simulink model "quadrotor_control"  (R2017b)
settings: Solver=FixedStepAuto  StartTime=0.0  StopTime=5  FixedStep=0.1  MinStep=0.02  RelTol=1e-3  AbsTol=0.001  EnableMultiTasking=on
PreLoadFcn:
  | m=0;
libraries: simulink x9
settings Model: Creator=GPH_PC  LastModifiedBy=dell
settings SolverCC: InitialStep=0.03
settings DataIOCC: LimitDataPoints=on  SaveFormat=Array
settings OptimizationCC: LifeSpan=inf
settings DebuggingCC: SolverPrmCheckMsg=warning  SFUnexpectedBacktrackingDiag=warning  SFNoUnconditionalDefaultTransitionDiag=warning  SFExecutionAtInitializationDiag=none
settings HardwareCC: ProdBitPerPointer=32  ProdBitPerSizeT=32  ProdBitPerPtrDiffT=32  ProdLargestAtomicFloat=None  ProdIntDivRoundTo=Undefined  ProdEndianess=Unspecified  ProdWordSize=32  ProdHWDeviceType=32-bit Generic
settings ModelReferenceCC: PropagateSignalLabelsOutOfModel=off
settings CodeAppCC: StateflowObjectComments=on
settings GRTTargetCC: TargetLangStandard=C89/C90 (ANSI)  GeneratePreprocessorConditionals=Disable all
settings ConfigComp: CovMetricSettings=dw  CovHtmlReporting=on  CovSaveCumulativeToWorkspaceVar=on  CovSaveSingleToWorkspaceVar=on  CovExternalEMLEnable=off  CovSFcnEnable=off

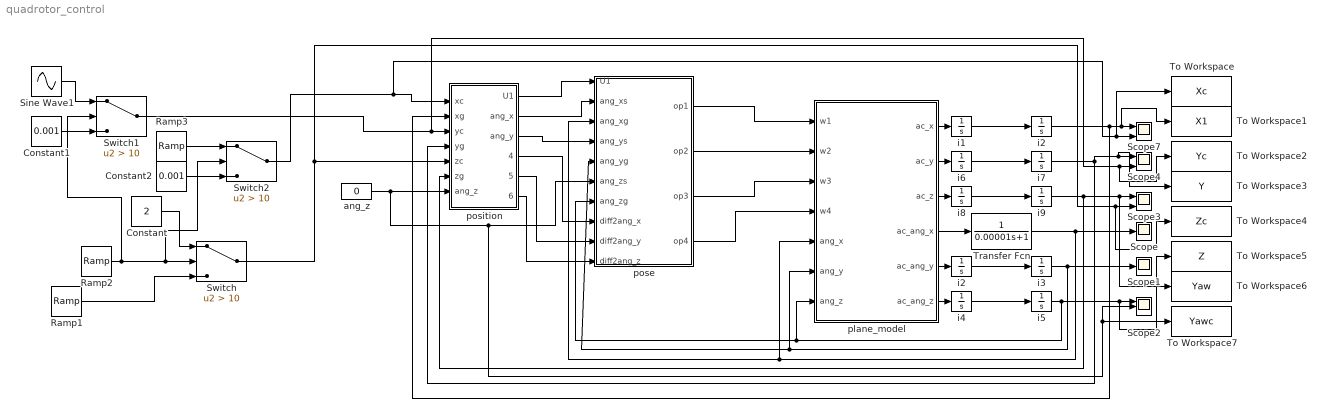
== system quadrotor_control ==
  " i2" : Integrator
  Constant : Constant  Value=2
  Constant1 : Constant  Value=0.001
  Constant2 : Constant  Value=0.001
  Ramp1 : simulink/Sources/Ramp  slope=0.2  start=0  X0=0
  Ramp2 : simulink/Sources/Ramp  slope=1  start=0  X0=0
  Ramp3 : simulink/Sources/Ramp  slope=1  start=0  X0=0
  Scope : Scope
  Scope1 : Scope
  Scope{2..4,7} (4 alike) : Scope  NumInputPorts=3
  Sine Wave1 : Sin  Amplitude=3  SampleTime=0
  Switch : Switch  Criteria=u2 > Threshold  Threshold=10
  Switch1 : Switch  Criteria=u2 > Threshold  Threshold=10
  Switch2 : Switch  Criteria=u2 > Threshold  Threshold=10
  To Workspace : ToWorkspace  VariableName=Xc  SampleTime=-1
      settings: Save2DSignal=2-D array (concatenate along first dimension)
  To Workspace1 : ToWorkspace  VariableName=X1  SampleTime=-1
      settings: Save2DSignal=2-D array (concatenate along first dimension)
  To Workspace2 : ToWorkspace  VariableName=Yc  SampleTime=-1
      settings: Save2DSignal=2-D array (concatenate along first dimension)
  To Workspace3 : ToWorkspace  VariableName=Y  SampleTime=-1
      settings: Save2DSignal=2-D array (concatenate along first dimension)
  To Workspace4 : ToWorkspace  VariableName=Zc  SampleTime=-1
      settings: Save2DSignal=2-D array (concatenate along first dimension)
  To Workspace5 : ToWorkspace  VariableName=Z  SampleTime=-1
      settings: Save2DSignal=2-D array (concatenate along first dimension)
  To Workspace6 : ToWorkspace  VariableName=Yaw  SampleTime=-1
      settings: Save2DSignal=2-D array (concatenate along first dimension)
  To Workspace7 : ToWorkspace  VariableName=Yawc  SampleTime=-1
      settings: Save2DSignal=2-D array (concatenate along first dimension)
  Transfer Fcn : TransferFcn  Numerator=[0 1]  Denominator=[0.00001 1]
  ang_z : Constant  Value=0
  i{1..9} (9 alike) : Integrator
  plane_model : MATLAB Function  TreatAsAtomicUnit=on
  pose : Subsystem
  position : Subsystem
  wires:
  pose/1(op1) -> plane_model/1(w1)
  pose/2(op2) -> plane_model/2(w2)
  pose/3(op3) -> plane_model/3(w3)
  pose/4(op4) -> plane_model/4(w4)
  i2/1 -> i3/1
  i4/1 -> i5/1
  plane_model/5(ac_ang_y) -> i2/1
  plane_model/6(ac_ang_z) -> i4/1
  i5/1 -> To Workspace6/1, Scope2/1, plane_model/7(ang_z), pose/7(ang_zg)
  i3/1 -> pose/5(ang_yg), plane_model/6(ang_y), Scope1/1
  Transfer Fcn/1 -> pose/3(ang_xg), plane_model/5(ang_x), Scope/1
  i1/1 -> " i2"/1
  i6/1 -> i7/1
  i8/1 -> i9/1
  plane_model/3(ac_z) -> i8/1
  plane_model/2(ac_y) -> i6/1
  plane_model/1(ac_x) -> i1/1
  i9/1 -> To Workspace5/1, Scope3/1, position/6(zg)
  i7/1 -> position/4(yg), To Workspace3/1, Scope4/1
  position/1(U1) -> pose/1(U1)
  position/3(ang_y) -> pose/4(ang_ys)
  ang_z/1 -> position/7(ang_z), To Workspace7/1, Scope2/2, pose/6(ang_zs)
  Switch/1 -> To Workspace4/1, Scope3/3, position/5(zc)
  Switch1/1 -> To Workspace2/1, Scope4/3, position/3(yc)
  Switch2/1 -> To Workspace/1, Scope7/3, position/1(xc)
  " i2"/1 -> To Workspace1/1, Scope7/1, position/2(xg)
  position/2(ang_x) -> pose/2(ang_xs)
  position/4(diff2 ang_x) -> pose/8(diff2ang_x)
  position/5(diff2 ang_y) -> pose/9(diff2ang_y)
  position/6(diff2 ang_z) -> pose/10(diff2ang_z)
  Ramp2/1 -> Switch1/2, Switch2/2, Switch/2
  Ramp1/1 -> Switch/3
  Constant/1 -> Switch/1
  Constant1/1 -> Switch1/3
  Sine Wave1/1 -> Switch1/1
  Ramp3/1 -> Switch2/1
  Constant2/1 -> Switch2/3
  plane_model/4(ac_ang_x) -> Transfer Fcn/1

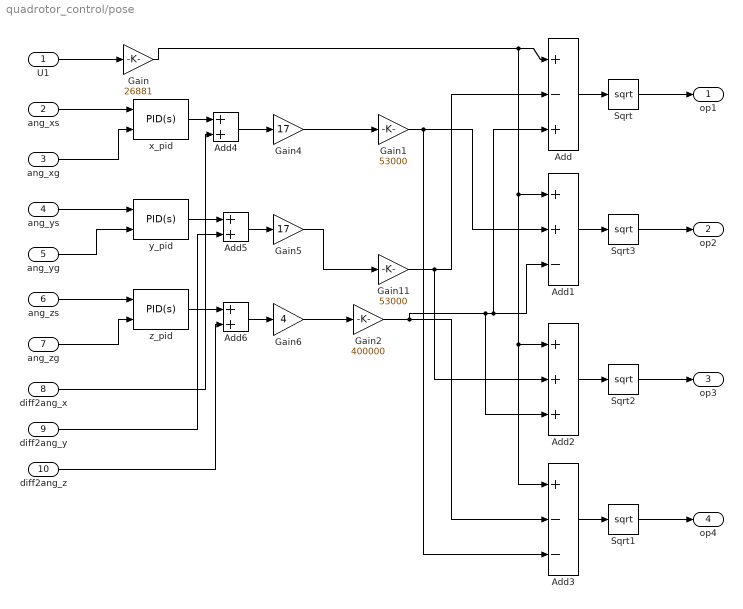
== system quadrotor_control/pose ==
  U1 : Inport
  ang_xs : Inport  Port=2
  ang_xg : Inport  Port=3
  ang_ys : Inport  Port=4
  ang_yg : Inport  Port=5
  ang_zs : Inport  Port=6
  ang_zg : Inport  Port=7
  diff2ang_x : Inport  Port=8
  diff2ang_y : Inport  Port=9
  diff2ang_z : Inport  Port=10
  Add : Sum  Inputs=+-+
  Add1 : Sum  Inputs=++-
  Add2 : Sum  Inputs=+++
  Add3 : Sum  Inputs=+--
  Add4 : Sum
  Add5 : Sum
  Add6 : Sum
  Gain : Gain  Gain=26881
  Gain1 : Gain  Gain=53000
  Gain11 : Gain  Gain=53000
  Gain2 : Gain  Gain=400000
  Gain4 : Gain  Gain=17
  Gain5 : Gain  Gain=17
  Gain6 : Gain  Gain=4
  Sqrt{,1..3} (4 alike) : Sqrt  SaturateOnIntegerOverflow=on
  x_pid : simulink/Continuous/PID Controller (2DOF)  Controller=PID  TimeDomain=Continuous-time  SampleTime=-1  IntegratorMethod=Forward Euler  FilterMethod=Forward Euler  Form=Parallel  UseFilter=on  ControllerParametersSource=internal  P=159  I=2  D=90  N=100  b=1  c=1  InitialConditionSource=internal  InitialConditionForIntegrator=0  InitialConditionForFilter=0  ExternalReset=none  LimitOutput=off  UpperSaturationLimit=inf  LowerSaturationLimit=-inf  LinearizeAsGain=on  AntiWindupMode=none  Kb=1  TrackingMode=off  Kt=1  PParamMin=[]  PParamMax=[]  IParamMin=[]  IParamMax=[]  DParamMin=[]  DParamMax=[]  NParamMin=[]  NParamMax=[]  bParamMin=[]  bParamMax=[]  cParamMin=[]  cParamMax=[]  KbParamMin=[]  KbParamMax=[]  KtParamMin=[]  KtParamMax=[]  POutMin=[]  POutMax=[]  IOutMin=[]  IOutMax=[]  DOutMin=[]  DOutMax=[]  NOutMin=[]  NOutMax=[]  bOutMin=[]  bOutMax=[]  cOutMin=[]  cOutMax=[]  KbOutMin=[]  KbOutMax=[]  KtOutMin=[]  KtOutMax=[]  IntegratorOutMin=[]  IntegratorOutMax=[]  FilterOutMin=[]  FilterOutMax=[]  SumOutMin=[]  SumOutMax=[]  Sum1OutMin=[]  Sum1OutMax=[]  Sum2OutMin=[]  Sum2OutMax=[]  Sum3OutMin=[]  Sum3OutMax=[]  SumI1OutMin=[]  SumI1OutMax=[]  SumI2OutMin=[]  SumI2OutMax=[]  SumI3OutMin=[]  SumI3OutMax=[]  SumDOutMin=[]  SumDOutMax=[]  SaturationOutMin=[]  SaturationOutMax=[]  IntegratorContinuousStateAttributes=''  IntegratorStateMustResolveToSignalObject=off  IntegratorRTWStateStorageClass=Auto  FilterContinuousStateAttributes=''  FilterStateMustResolveToSignalObject=off  FilterRTWStateStorageClass=Auto  DifferentiatorICPrevScaledInput=0  DifferentiatorOutMin=[]  DifferentiatorOutMax=[]  InitialConditionSetting=State (most efficient)  FilterDiffOutCoefMin=[]  FilterDiffOutCoefMax=[]  SumDenOutMin=[]  SumDenOutMax=[]  SumNumOutMin=[]  SumNumOutMax=[]  ReciprocalOutMin=[]  ReciprocalOutMax=[]  DivideOutMin=[]  DivideOutMax=[]  TunerSelectOption=Transfer Function Based (PID Tuner App)
  y_pid : simulink/Continuous/PID Controller (2DOF)  Controller=PID  TimeDomain=Continuous-time  SampleTime=-1  IntegratorMethod=Forward Euler  FilterMethod=Forward Euler  Form=Parallel  UseFilter=on  ControllerParametersSource=internal  P=150  I=2  D=90  N=100  b=1  c=1  InitialConditionSource=internal  InitialConditionForIntegrator=0  InitialConditionForFilter=0  ExternalReset=none  LimitOutput=off  UpperSaturationLimit=inf  LowerSaturationLimit=-inf  LinearizeAsGain=on  AntiWindupMode=none  Kb=1  TrackingMode=off  Kt=1  PParamMin=[]  PParamMax=[]  IParamMin=[]  IParamMax=[]  DParamMin=[]  DParamMax=[]  NParamMin=[]  NParamMax=[]  bParamMin=[]  bParamMax=[]  cParamMin=[]  cParamMax=[]  KbParamMin=[]  KbParamMax=[]  KtParamMin=[]  KtParamMax=[]  POutMin=[]  POutMax=[]  IOutMin=[]  IOutMax=[]  DOutMin=[]  DOutMax=[]  NOutMin=[]  NOutMax=[]  bOutMin=[]  bOutMax=[]  cOutMin=[]  cOutMax=[]  KbOutMin=[]  KbOutMax=[]  KtOutMin=[]  KtOutMax=[]  IntegratorOutMin=[]  IntegratorOutMax=[]  FilterOutMin=[]  FilterOutMax=[]  SumOutMin=[]  SumOutMax=[]  Sum1OutMin=[]  Sum1OutMax=[]  Sum2OutMin=[]  Sum2OutMax=[]  Sum3OutMin=[]  Sum3OutMax=[]  SumI1OutMin=[]  SumI1OutMax=[]  SumI2OutMin=[]  SumI2OutMax=[]  SumI3OutMin=[]  SumI3OutMax=[]  SumDOutMin=[]  SumDOutMax=[]  SaturationOutMin=[]  SaturationOutMax=[]  IntegratorContinuousStateAttributes=''  IntegratorStateMustResolveToSignalObject=off  IntegratorRTWStateStorageClass=Auto  FilterContinuousStateAttributes=''  FilterStateMustResolveToSignalObject=off  FilterRTWStateStorageClass=Auto  DifferentiatorICPrevScaledInput=0  DifferentiatorOutMin=[]  DifferentiatorOutMax=[]  InitialConditionSetting=State (most efficient)  FilterDiffOutCoefMin=[]  FilterDiffOutCoefMax=[]  SumDenOutMin=[]  SumDenOutMax=[]  SumNumOutMin=[]  SumNumOutMax=[]  ReciprocalOutMin=[]  ReciprocalOutMax=[]  DivideOutMin=[]  DivideOutMax=[]  TunerSelectOption=Transfer Function Based (PID Tuner App)
  z_pid : simulink/Continuous/PID Controller (2DOF)  Controller=PID  TimeDomain=Continuous-time  SampleTime=-1  IntegratorMethod=Forward Euler  FilterMethod=Forward Euler  Form=Parallel  UseFilter=on  ControllerParametersSource=internal  P=10  I=0  D=20  N=100  b=1  c=1  InitialConditionSource=internal  InitialConditionForIntegrator=0  InitialConditionForFilter=0  ExternalReset=none  LimitOutput=off  UpperSaturationLimit=inf  LowerSaturationLimit=-inf  LinearizeAsGain=on  AntiWindupMode=none  Kb=1  TrackingMode=off  Kt=1  PParamMin=[]  PParamMax=[]  IParamMin=[]  IParamMax=[]  DParamMin=[]  DParamMax=[]  NParamMin=[]  NParamMax=[]  bParamMin=[]  bParamMax=[]  cParamMin=[]  cParamMax=[]  KbParamMin=[]  KbParamMax=[]  KtParamMin=[]  KtParamMax=[]  POutMin=[]  POutMax=[]  IOutMin=[]  IOutMax=[]  DOutMin=[]  DOutMax=[]  NOutMin=[]  NOutMax=[]  bOutMin=[]  bOutMax=[]  cOutMin=[]  cOutMax=[]  KbOutMin=[]  KbOutMax=[]  KtOutMin=[]  KtOutMax=[]  IntegratorOutMin=[]  IntegratorOutMax=[]  FilterOutMin=[]  FilterOutMax=[]  SumOutMin=[]  SumOutMax=[]  Sum1OutMin=[]  Sum1OutMax=[]  Sum2OutMin=[]  Sum2OutMax=[]  Sum3OutMin=[]  Sum3OutMax=[]  SumI1OutMin=[]  SumI1OutMax=[]  SumI2OutMin=[]  SumI2OutMax=[]  SumI3OutMin=[]  SumI3OutMax=[]  SumDOutMin=[]  SumDOutMax=[]  SaturationOutMin=[]  SaturationOutMax=[]  IntegratorContinuousStateAttributes=''  IntegratorStateMustResolveToSignalObject=off  IntegratorRTWStateStorageClass=Auto  FilterContinuousStateAttributes=''  FilterStateMustResolveToSignalObject=off  FilterRTWStateStorageClass=Auto  DifferentiatorICPrevScaledInput=0  DifferentiatorOutMin=[]  DifferentiatorOutMax=[]  InitialConditionSetting=State (most efficient)  FilterDiffOutCoefMin=[]  FilterDiffOutCoefMax=[]  SumDenOutMin=[]  SumDenOutMax=[]  SumNumOutMin=[]  SumNumOutMax=[]  ReciprocalOutMin=[]  ReciprocalOutMax=[]  DivideOutMin=[]  DivideOutMax=[]  TunerSelectOption=Transfer Function Based (PID Tuner App)
  op1 : Outport
  op2 : Outport  Port=2
  op3 : Outport  Port=3
  op4 : Outport  Port=4
  wires:
  U1/1 -> Gain/1
  Gain/1 -> Add3/1, Add2/1, Add1/1, Add/1
  ang_ys/1 -> y_pid/1
  ang_yg/1 -> y_pid/2
  ang_xs/1 -> x_pid/1
  ang_xg/1 -> x_pid/2
  ang_zs/1 -> z_pid/1
  ang_zg/1 -> z_pid/2
  x_pid/1 -> Add4/1
  diff2ang_x/1 -> Add4/2
  y_pid/1 -> Add5/1
  diff2ang_y/1 -> Add5/2
  z_pid/1 -> Add6/1
  diff2ang_z/1 -> Add6/2
  Add4/1 -> Gain4/1
  Add5/1 -> Gain5/1
  Add6/1 -> Gain6/1
  Add/1 -> Sqrt/1
  Gain6/1 -> Gain2/1
  Gain2/1 -> Add2/3, Add/3, Add1/3, Add3/2
  Gain4/1 -> Gain1/1
  Gain5/1 -> Gain11/1
  Gain11/1 -> Add2/2, Add/2
  Gain1/1 -> Add3/3, Add1/2
  Sqrt/1 -> op1/1
  Add1/1 -> Sqrt3/1
  Sqrt3/1 -> op2/1
  Add2/1 -> Sqrt2/1
  Sqrt2/1 -> op3/1
  Add3/1 -> Sqrt1/1
  Sqrt1/1 -> op4/1

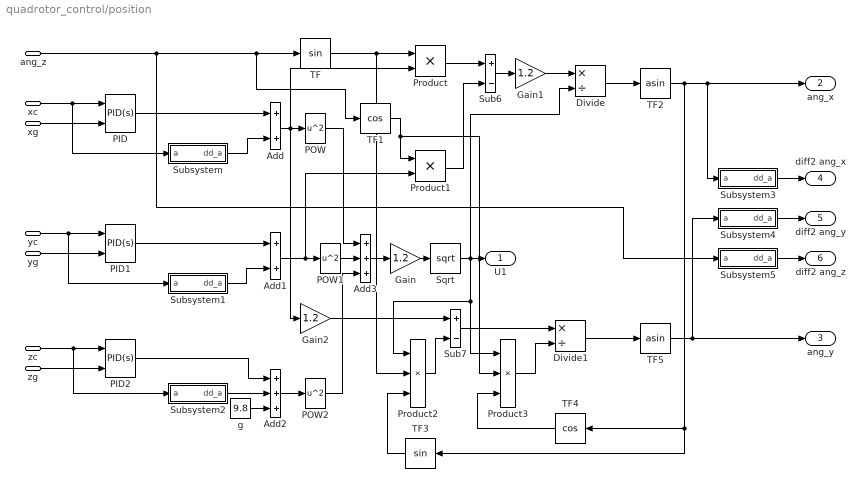
== system quadrotor_control/position ==
  xc : Inport
  xg : Inport  Port=2
  yc : Inport  Port=3
  yg : Inport  Port=4
  zc : Inport  Port=5
  zg : Inport  Port=6
  ang_z : Inport  Port=7
  Add : Sum
  Add1 : Sum
  Add2 : Sum  Inputs=+++
  Add3 : Sum  Inputs=+++
  Divide : Product  Inputs=*/
  Divide1 : Product  Inputs=*/
  Gain : Gain  Gain=1.2
  Gain1 : Gain  Gain=1.2
  Gain2 : Gain  Gain=1.2
  PID : simulink/Continuous/PID Controller (2DOF)  Controller=PID  TimeDomain=Continuous-time  SampleTime=-1  IntegratorMethod=Forward Euler  FilterMethod=Forward Euler  Form=Parallel  UseFilter=on  ControllerParametersSource=internal  P=70  I=5  D=75  N=100  b=1  c=1  InitialConditionSource=internal  InitialConditionForIntegrator=0  InitialConditionForFilter=0  ExternalReset=none  LimitOutput=off  UpperSaturationLimit=inf  LowerSaturationLimit=-inf  LinearizeAsGain=on  AntiWindupMode=none  Kb=1  TrackingMode=off  Kt=1  PParamMin=[]  PParamMax=[]  IParamMin=[]  IParamMax=[]  DParamMin=[]  DParamMax=[]  NParamMin=[]  NParamMax=[]  bParamMin=[]  bParamMax=[]  cParamMin=[]  cParamMax=[]  KbParamMin=[]  KbParamMax=[]  KtParamMin=[]  KtParamMax=[]  POutMin=[]  POutMax=[]  IOutMin=[]  IOutMax=[]  DOutMin=[]  DOutMax=[]  NOutMin=[]  NOutMax=[]  bOutMin=[]  bOutMax=[]  cOutMin=[]  cOutMax=[]  KbOutMin=[]  KbOutMax=[]  KtOutMin=[]  KtOutMax=[]  IntegratorOutMin=[]  IntegratorOutMax=[]  FilterOutMin=[]  FilterOutMax=[]  SumOutMin=[]  SumOutMax=[]  Sum1OutMin=[]  Sum1OutMax=[]  Sum2OutMin=[]  Sum2OutMax=[]  Sum3OutMin=[]  Sum3OutMax=[]  SumI1OutMin=[]  SumI1OutMax=[]  SumI2OutMin=[]  SumI2OutMax=[]  SumI3OutMin=[]  SumI3OutMax=[]  SumDOutMin=[]  SumDOutMax=[]  SaturationOutMin=[]  SaturationOutMax=[]  IntegratorContinuousStateAttributes=''  IntegratorStateMustResolveToSignalObject=off  IntegratorRTWStateStorageClass=Auto  FilterContinuousStateAttributes=''  FilterStateMustResolveToSignalObject=off  FilterRTWStateStorageClass=Auto  DifferentiatorICPrevScaledInput=0  DifferentiatorOutMin=[]  DifferentiatorOutMax=[]  InitialConditionSetting=State (most efficient)  FilterDiffOutCoefMin=[]  FilterDiffOutCoefMax=[]  SumDenOutMin=[]  SumDenOutMax=[]  SumNumOutMin=[]  SumNumOutMax=[]  ReciprocalOutMin=[]  ReciprocalOutMax=[]  DivideOutMin=[]  DivideOutMax=[]  TunerSelectOption=Transfer Function Based (PID Tuner App)
  PID1 : simulink/Continuous/PID Controller (2DOF)  Controller=PID  TimeDomain=Continuous-time  SampleTime=-1  IntegratorMethod=Forward Euler  FilterMethod=Forward Euler  Form=Parallel  UseFilter=on  ControllerParametersSource=internal  P=75  I=5  D=75  N=100  b=1  c=1  InitialConditionSource=internal  InitialConditionForIntegrator=0  InitialConditionForFilter=0  ExternalReset=none  LimitOutput=off  UpperSaturationLimit=inf  LowerSaturationLimit=-inf  LinearizeAsGain=on  AntiWindupMode=none  Kb=1  TrackingMode=off  Kt=1  PParamMin=[]  PParamMax=[]  IParamMin=[]  IParamMax=[]  DParamMin=[]  DParamMax=[]  NParamMin=[]  NParamMax=[]  bParamMin=[]  bParamMax=[]  cParamMin=[]  cParamMax=[]  KbParamMin=[]  KbParamMax=[]  KtParamMin=[]  KtParamMax=[]  POutMin=[]  POutMax=[]  IOutMin=[]  IOutMax=[]  DOutMin=[]  DOutMax=[]  NOutMin=[]  NOutMax=[]  bOutMin=[]  bOutMax=[]  cOutMin=[]  cOutMax=[]  KbOutMin=[]  KbOutMax=[]  KtOutMin=[]  KtOutMax=[]  IntegratorOutMin=[]  IntegratorOutMax=[]  FilterOutMin=[]  FilterOutMax=[]  SumOutMin=[]  SumOutMax=[]  Sum1OutMin=[]  Sum1OutMax=[]  Sum2OutMin=[]  Sum2OutMax=[]  Sum3OutMin=[]  Sum3OutMax=[]  SumI1OutMin=[]  SumI1OutMax=[]  SumI2OutMin=[]  SumI2OutMax=[]  SumI3OutMin=[]  SumI3OutMax=[]  SumDOutMin=[]  SumDOutMax=[]  SaturationOutMin=[]  SaturationOutMax=[]  IntegratorContinuousStateAttributes=''  IntegratorStateMustResolveToSignalObject=off  IntegratorRTWStateStorageClass=Auto  FilterContinuousStateAttributes=''  FilterStateMustResolveToSignalObject=off  FilterRTWStateStorageClass=Auto  DifferentiatorICPrevScaledInput=0  DifferentiatorOutMin=[]  DifferentiatorOutMax=[]  InitialConditionSetting=State (most efficient)  FilterDiffOutCoefMin=[]  FilterDiffOutCoefMax=[]  SumDenOutMin=[]  SumDenOutMax=[]  SumNumOutMin=[]  SumNumOutMax=[]  ReciprocalOutMin=[]  ReciprocalOutMax=[]  DivideOutMin=[]  DivideOutMax=[]  TunerSelectOption=Transfer Function Based (PID Tuner App)
  PID2 : simulink/Continuous/PID Controller (2DOF)  Controller=PID  TimeDomain=Continuous-time  SampleTime=-1  IntegratorMethod=Forward Euler  FilterMethod=Forward Euler  Form=Parallel  UseFilter=on  ControllerParametersSource=internal  P=200  I=75  D=100  N=100  b=1  c=1  InitialConditionSource=internal  InitialConditionForIntegrator=0  InitialConditionForFilter=0  ExternalReset=none  LimitOutput=off  UpperSaturationLimit=inf  LowerSaturationLimit=-inf  LinearizeAsGain=on  AntiWindupMode=none  Kb=1  TrackingMode=off  Kt=1  PParamMin=[]  PParamMax=[]  IParamMin=[]  IParamMax=[]  DParamMin=[]  DParamMax=[]  NParamMin=[]  NParamMax=[]  bParamMin=[]  bParamMax=[]  cParamMin=[]  cParamMax=[]  KbParamMin=[]  KbParamMax=[]  KtParamMin=[]  KtParamMax=[]  POutMin=[]  POutMax=[]  IOutMin=[]  IOutMax=[]  DOutMin=[]  DOutMax=[]  NOutMin=[]  NOutMax=[]  bOutMin=[]  bOutMax=[]  cOutMin=[]  cOutMax=[]  KbOutMin=[]  KbOutMax=[]  KtOutMin=[]  KtOutMax=[]  IntegratorOutMin=[]  IntegratorOutMax=[]  FilterOutMin=[]  FilterOutMax=[]  SumOutMin=[]  SumOutMax=[]  Sum1OutMin=[]  Sum1OutMax=[]  Sum2OutMin=[]  Sum2OutMax=[]  Sum3OutMin=[]  Sum3OutMax=[]  SumI1OutMin=[]  SumI1OutMax=[]  SumI2OutMin=[]  SumI2OutMax=[]  SumI3OutMin=[]  SumI3OutMax=[]  SumDOutMin=[]  SumDOutMax=[]  SaturationOutMin=[]  SaturationOutMax=[]  IntegratorContinuousStateAttributes=''  IntegratorStateMustResolveToSignalObject=off  IntegratorRTWStateStorageClass=Auto  FilterContinuousStateAttributes=''  FilterStateMustResolveToSignalObject=off  FilterRTWStateStorageClass=Auto  DifferentiatorICPrevScaledInput=0  DifferentiatorOutMin=[]  DifferentiatorOutMax=[]  InitialConditionSetting=State (most efficient)  FilterDiffOutCoefMin=[]  FilterDiffOutCoefMax=[]  SumDenOutMin=[]  SumDenOutMax=[]  SumNumOutMin=[]  SumNumOutMax=[]  ReciprocalOutMin=[]  ReciprocalOutMax=[]  DivideOutMin=[]  DivideOutMax=[]  TunerSelectOption=Transfer Function Based (PID Tuner App)
  POW : Math  Operator=square  SaturateOnIntegerOverflow=on
  POW1 : Math  Operator=square  SaturateOnIntegerOverflow=on
  POW2 : Math  Operator=square  SaturateOnIntegerOverflow=on
  Product : Product
  Product1 : Product
  Product2 : Product  Inputs=3
  Product3 : Product  Inputs=3
  Sqrt : Sqrt  SaturateOnIntegerOverflow=on
  Sub6 : Sum  Inputs=+-
  Sub7 : Sum  Inputs=+-
  Subsystem : Subsystem
  Subsystem1 : Subsystem
  Subsystem2 : Subsystem
  Subsystem3 : Subsystem
  Subsystem4 : Subsystem
  Subsystem5 : Subsystem
  TF : Trigonometry
  TF1 : Trigonometry  Operator=cos
  TF2 : Trigonometry  Operator=asin
  TF3 : Trigonometry
  TF4 : Trigonometry  Operator=cos
  TF5 : Trigonometry  Operator=asin
  g : Constant  Value=9.8
  U1 : Outport
  ang_x : Outport  Port=2
  ang_y : Outport  Port=3
  diff2 ang_x : Outport  Port=4
  diff2 ang_y : Outport  Port=5
  diff2 ang_z : Outport  Port=6
  wires:
  Add/1 -> Gain2/1, Product/2, POW/1
  Add1/1 -> Product1/2, POW1/1
  g/1 -> Add2/3
  Add2/1 -> POW2/1
  POW1/1 -> Add3/2
  POW/1 -> Add3/1
  POW2/1 -> Add3/3
  Add3/1 -> Gain/1
  Gain/1 -> Sqrt/1
  Sqrt/1 -> Product3/1, Product2/1, Divide/2, U1/1
  ang_z/1 -> Subsystem5/1(a), TF1/1, TF/1
  TF/1 -> Product/1, Product2/2
  Product/1 -> Sub6/1
  TF1/1 -> Product1/1, Product3/2
  Product1/1 -> Sub6/2
  Sub6/1 -> Gain1/1
  Gain1/1 -> Divide/1
  Divide/1 -> TF2/1
  TF2/1 -> TF4/1, TF3/1, Subsystem3/1(a), ang_x/1
  Gain2/1 -> Sub7/1
  Product2/1 -> Sub7/2
  Sub7/1 -> Divide1/1
  TF3/1 -> Product2/3
  TF4/1 -> Product3/3
  Product3/1 -> Divide1/2
  Divide1/1 -> TF5/1
  TF5/1 -> Subsystem4/1(a), ang_y/1
  xc/1 -> Subsystem/1(a), PID/1
  xg/1 -> PID/2
  PID/1 -> Add/1
  Subsystem/1(dd_a) -> Add/2
  yc/1 -> Subsystem1/1(a), PID1/1
  yg/1 -> PID1/2
  PID1/1 -> Add1/1
  Subsystem1/1(dd_a) -> Add1/2
  Subsystem2/1(dd_a) -> Add2/2
  PID2/1 -> Add2/1
  zc/1 -> Subsystem2/1(a), PID2/1
  zg/1 -> PID2/2
  Subsystem3/1(dd_a) -> diff2 ang_x/1
  Subsystem5/1(dd_a) -> diff2 ang_z/1
  Subsystem4/1(dd_a) -> diff2 ang_y/1

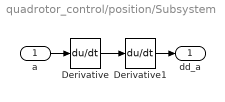
== system quadrotor_control/position/Subsystem ==
  a : Inport
  Derivative : Derivative
  Derivative1 : Derivative
  dd_a : Outport
  wires:
  Derivative1/1 -> dd_a/1
  a/1 -> Derivative/1
  Derivative/1 -> Derivative1/1

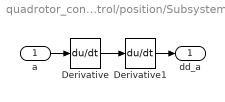
== system quadrotor_control/position/Subsystem1 ==
  a : Inport
  Derivative : Derivative
  Derivative1 : Derivative
  dd_a : Outport
  wires:
  Derivative1/1 -> dd_a/1
  a/1 -> Derivative/1
  Derivative/1 -> Derivative1/1

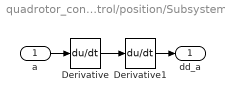
== system quadrotor_control/position/Subsystem2 ==
  a : Inport
  Derivative : Derivative
  Derivative1 : Derivative
  dd_a : Outport
  wires:
  Derivative1/1 -> dd_a/1
  a/1 -> Derivative/1
  Derivative/1 -> Derivative1/1

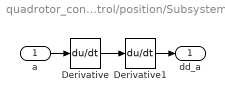
== system quadrotor_control/position/Subsystem3 ==
  a : Inport
  Derivative : Derivative
  Derivative1 : Derivative
  dd_a : Outport
  wires:
  Derivative1/1 -> dd_a/1
  a/1 -> Derivative/1
  Derivative/1 -> Derivative1/1

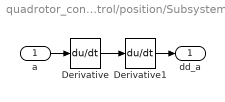
== system quadrotor_control/position/Subsystem4 ==
  a : Inport
  Derivative : Derivative
  Derivative1 : Derivative
  dd_a : Outport
  wires:
  Derivative1/1 -> dd_a/1
  a/1 -> Derivative/1
  Derivative/1 -> Derivative1/1

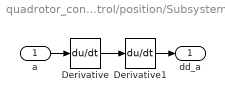
== system quadrotor_control/position/Subsystem5 ==
  a : Inport
  Derivative : Derivative
  Derivative1 : Derivative
  dd_a : Outport
  wires:
  Derivative1/1 -> dd_a/1
  a/1 -> Derivative/1
  Derivative/1 -> Derivative1/1

== matlab function quadrotor_control/plane_model ==
  data: w1 input; ac_x output; w2 input; w3 input; w4 input; ac_y output; ac_z output; ac_ang_x output; ac_ang_y output; ac_ang_z output; ang_x input; ang_y input; ang_z input
function [ac_x,ac_y,ac_z,ac_ang_x,ac_ang_y,ac_ang_z] = fcn(w1,w2,w3,w4,ang_x,ang_y,ang_z)
%#codegen
kb=3.1e-5;Ix=17.333;Iy=17.33;Iz=4.33;m=1.2;kt=2.1e-6;L=0.3;
U1=kb*(w1*w1+w2*w2+w3*w3+w4*w4)*L;
U2=kb*(w2*w2-w4*w4)*L;
U3=kb*(w3*w3-w1*w1)*L;
U4=kt*(w1*w1+w3*w3-w2*w2-w4*w4)*L;
ac_x=U1*(sin(ang_x)*sin(ang_z)+cos(ang_z)*sin(ang_y)*cos(ang_x))/m;
ac_y=U1*(sin(ang_z)*sin(ang_y)*cos(ang_x)-cos(ang_z)*sin(ang_x))/m;
ac_z=U1*cos(ang_x)*cos(ang_y)/m-9.8;
ac_ang_x=U2*Ix;
ac_ang_y=U3*Iy; 
ac_ang_z=U4*Iz;
